simulink model "MPCQP"  (R2025b)
settings: Solver=ode14x  StartTime=0.0  StopTime=10.0  FixedStep=Ts_local  RelTol=1e-3
model workspace (MAT data in the model file):
  A = [0.885698933699 -0.394986604769 -0.0779918473435 0.0101055350413 0.00217449311718 -0.00926746047024 -8.99143110462e-05 0.00234447011447 -0.0164960253387 -0.00706632129504 0.0082006041579 -0.0223008473046 ... (196 elements, 14x14)]
  B = [-0.0512463384039  -0.0611116643133  -0.111555539394; -0.234744164447  -0.312351229732  -0.865399165809; -0.540554485725  -0.953035386549  -2.17092555742; -0.20088655759  -0.169711047475  0.210134088405; -0.248357104431  -0.857338100977  0.331995476801; -1.79033982746  -1.38369463415  0.683809798908; -0.12549830699  -0.578244159563  0.253779209638; 0.405207526436  -0.410231528068  0.18915279719; -1.65577071746  1.4613881888  -0.525385297952; -0.608655393628  -0.904593475383  0.76373521164; -1.1672857761  0.132715605127  -0.776223165643; -0.210779013302  0.990283180789  0.753402996085; 0.255866591317  0.15454031663  0.481591109924; 0.172174296523  -0.147203742515  0.591060823112]
  C = [0.000135237526108  0.000106430205441  -1.41257234742e-05  0.000636797939839  0.00111774077127  0.00093714511309  -0.00129418331211  -0.0028438157941  0.000395173743571  -0.00131691652412  -0.00236174719739  -0.00100478778794  5.77955970205e-06  -0.000114759416285; 0.000386710765865  0.000986636703051  0.000214883313837  0.00140638779609  0.00302801539836  -0.000204365156932  0.000640359779749  0.00155096708917  -0.000168323329419  -0.0021734439855  0.000518036248978  0.00233701888615  -4.04586319889e-05  -3.62969428899e-05; 0.00161442227176  0.00388504471451  0.000329789732914  -0.000872629917614  -0.00131408872479  -0.000395145603667  0.000190410605135  0.000609064188035  -0.000123048402414  0.00235557919401  -0.00129025398477  0.0026831376772  3.92692859894e-05  0.000133299695507]
  D = [0  0  0; 0  0  0; 0  0  0]
  L = [0.404810109514  1.70785067155  1.21319355104; 2.21427010781  -0.745616724697  -1.94972006746; -1.48829714444  8.79874280294  5.92032601042; 9.02503127585  6.61002508707  -2.91974304326; -10.3205357615  -7.67253560184  1.54884946757; 47.9226177365  25.8586998172  -12.9349454943; -6.05718994132  16.1956236822  -3.01213767158; 22.0543247881  -6.77966289631  -1.62335098876; 39.0442082476  -45.0455727297  1.57847873955; -134.695110952  -226.113610754  147.134904861; -328.93545888  36.0630667452  -158.542396292; -42.5648255842  213.488675601  171.017168568; 55.5332402883  20.6569204967  -93.4344140149; -16.9970193503  61.6508931048  18.4048062569]
  N1 = 1
  N2 = 20
  Nu = 10
  alpha = [0.2 0.2 0.2]
  du_init = [0 0 0]
  dumax = [inf inf inf]
  dumin = [-inf -inf -inf]
  lam = [1 1 1]
  solve_when_inactive = 0
  u_init = [0 0 0]
  umax = [0.1579 0.1579 0.1579]
  umin = [-0.3612 -0.3612 -0.3612]
  use_quadprog = 1
  wy = [10 10 10]
values from neighbouring files (symbols this model uses):
  Ts_ctrl = 0.1    [ctrlSys.sldd]
settings Model: DataDictionary=ctrlSys.sldd  Creator=LYG  LastModifiedBy=LYG

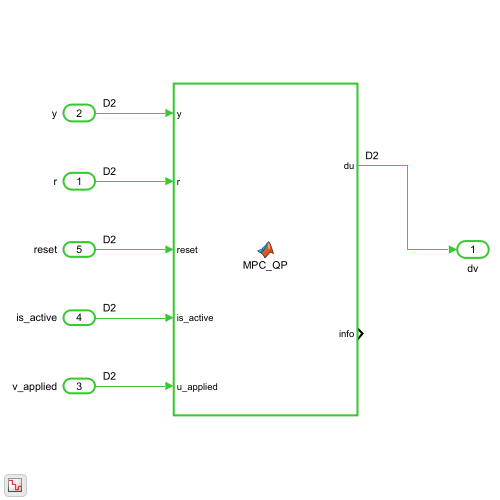
[thumbnail: Simulink's stored preview of the top-level diagram]
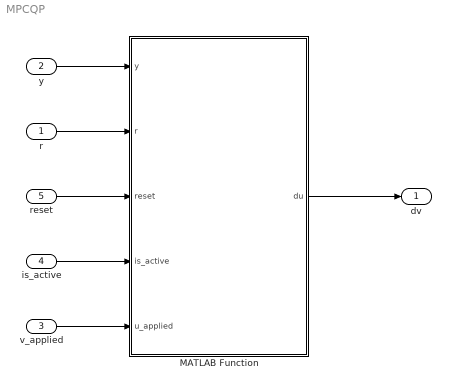
== system MPCQP ==
  r : Inport
  y : Inport  Port=2
  v_applied : Inport  Port=3
  is_active : Inport  Port=4
  reset : Inport  Port=5
  MATLAB Function : MATLAB Function  TreatAsAtomicUnit=on  SystemSampleTime=Ts_ctrl
  dv : Outport
  wires:
  r/1 -> MATLAB Function/2(r)
  reset/1 -> MATLAB Function/3(reset)
  y/1 -> MATLAB Function/1(y)
  v_applied/1 -> MATLAB Function/5(u_applied)
  is_active/1 -> MATLAB Function/4(is_active)
  MATLAB Function/1(du) -> dv/1

== matlab function MPCQP/MATLAB Function ==
  data: y input size=[3 1]; du output size=[3 1]; r input size=[3 1]; A parameter; B parameter; N1 parameter size=[1 1]; N2 parameter size=[1 1]; Nu parameter size=[1 1]; alpha parameter; lam parameter; reset input size=[1 1]; C parameter; D parameter; wy parameter; umin parameter; umax parameter; dumin parameter; dumax parameter; u_init parameter; du_init parameter; L parameter; use_quadprog parameter size=[1 1]; is_active input boolean size=[1 1]; u_applied input size=[3 1]; solve_when_inactive parameter size=[1 1]
function du = MPC_QP(y, r, A, B, N1, N2, Nu, alpha, lam, reset, ...
                    C, D, wy, umin, umax, dumin, dumax, u_init, du_init, ...
                    L, use_quadprog, is_active, u_applied, solve_when_inactive)
%MPC_QP Constrained MPC wrapper with optional supervisor inputs.
%   This wrapper preserves the public MATLAB entry point and delegates the
%   implementation to MPC_QP_core so Simulink and script callers can share
%   the same controller logic.

    if nargout > 1
        if nargin == 21
            [du, info] = MPC_QP_core(y, r, A, B, N1, N2, Nu, alpha, lam, reset, ...
                                     C, D, wy, umin, umax, dumin, dumax, u_init, du_init, ...
                                     L, use_quadprog);
        elseif nargin == 22
            [du, info] = MPC_QP_core(y, r, A, B, N1, N2, Nu, alpha, lam, reset, ...
                                     C, D, wy, umin, umax, dumin, dumax, u_init, du_init, ...
                                     L, use_quadprog, is_active);
        elseif nargin == 23
            [du, info] = MPC_QP_core(y, r, A, B, N1, N2, Nu, alpha, lam, reset, ...
                                     C, D, wy, umin, umax, dumin, dumax, u_init, du_init, ...
                                     L, use_quadprog, is_active, u_applied);
        else
            [du, info] = MPC_QP_core(y, r, A, B, N1, N2, Nu, alpha, lam, reset, ...
                                     C, D, wy, umin, umax, dumin, dumax, u_init, du_init, ...
                                     L, use_quadprog, is_active, u_applied, solve_when_inactive);
        end
    else
        if nargin == 21
            du = MPC_QP_core(y, r, A, B, N1, N2, Nu, alpha, lam, reset, ...
                             C, D, wy, umin, umax, dumin, dumax, u_init, du_init, ...
                             L, use_quadprog);
        elseif nargin == 22
            du = MPC_QP_core(y, r, A, B, N1, N2, Nu, alpha, lam, reset, ...
                             C, D, wy, umin, umax, dumin, dumax, u_init, du_init, ...
                             L, use_quadprog, is_active);
        elseif nargin == 23
            du = MPC_QP_core(y, r, A, B, N1, N2, Nu, alpha, lam, reset, ...
                             C, D, wy, umin, umax, dumin, dumax, u_init, du_init, ...
                             L, use_quadprog, is_active, u_applied);
        else
            du = MPC_QP_core(y, r, A, B, N1, N2, Nu, alpha, lam, reset, ...
                             C, D, wy, umin, umax, dumin, dumax, u_init, du_init, ...
                             L, use_quadprog, is_active, u_applied, solve_when_inactive);
        end
    end
end
